simulink model "mmr_air_backup"  (R2019a)
settings: Solver=VariableStepAuto  StartTime=0.0  StopTime=ta  RelTol=1e-1
values from neighbouring files (symbols this model uses):
  g = -9.81    [MMR.m]    (also in MMR_alfa0.m; MMR_alone.m; MMR_hop_zero.m = 9.81)
  Lcol = 0.70    (= 0.7)    [MMR.m]    (also in MMR_alone.m)
  Lhk = 0.28    [MMR.m]    (also in MMR_alfa0.m; MMR_alone.m; MMR_hop_zero.m)
  Lkf = 0.28    [MMR.m]    (also in MMR_alfa0.m; MMR_alone.m; MMR_hop_zero.m)
  M = 15    [MMR.m]    (also in MMR_alfa0.m; MMR_alone.m; MMR_hop_zero.m)
  m = 3    [MMR.m]    (also in MMR_alfa0.m; MMR_alone.m; MMR_hop_zero.m)
  vxfinal = vx( length(vx) )    [MMR.m]    (also in MMR_alfa0.m; MMR_alone.m)
  vxMfinal = vxM( length(vxM) )    [MMR.m]    (also in MMR_alfa0.m; MMR_alone.m)
  vyfinal = vy( length(vy) )    [MMR.m]    (also in MMR_alfa0.m; MMR_alone.m; MMR_hop_zero.m)
  vyMfinal = vyM( length(vyM) )    [MMR.m]    (also in MMR_alfa0.m; MMR_alone.m)
  xfinal = x( length(x) )    [MMR.m]    (also in MMR_alfa0.m; MMR_alone.m)
  xMfinal = xM( length(xM) )    [MMR.m]    (also in MMR_alfa0.m; MMR_alone.m)
  yfinal = y( length(y) )    [MMR.m]    (also in MMR_alfa0.m; MMR_alone.m; MMR_hop_zero.m)
  yMfinal = yM( length(yM) )    [MMR.m]    (also in MMR_alfa0.m; MMR_alone.m)
undefined symbols (not defined in the file or in its folder): magnitude
settings Model: Creator=Jesus  LastModifiedBy=Jesus

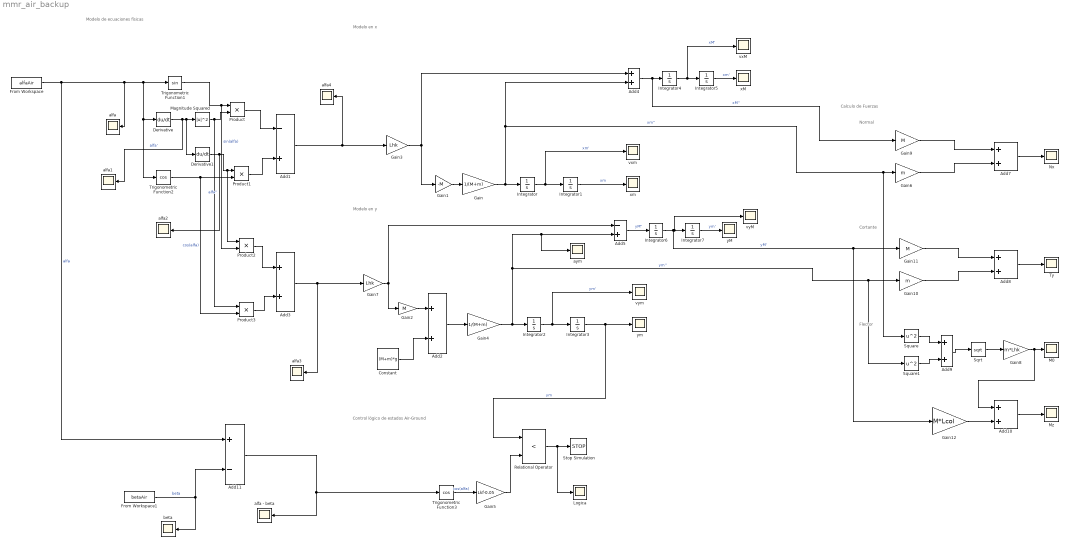
== system mmr_air_backup ==
  note: Control lógico de estados Air-Ground
  note: Modelo de ecuaciones físicas
  note: Modelo en x
  note: Modelo en y
  note: Calculo de Fuerzas
  note: Normal
  note: Cortante
  note: Flector
  Add1 : Sum  Inputs=-+
  Add{2..4,7..10} (7 alike) : Sum
  Add11 : Sum  Inputs=+-
  Add5 : Sum  Inputs=-+
  Constant : Constant  Value=(M+m)*g
  Derivative : Derivative  CoefficientInTFapproximation=1000
  Derivative1 : Derivative  CoefficientInTFapproximation=1000
  From Workspace : FromWorkspace  VariableName=alfaAir  SampleTime=0
  From Workspace1 : FromWorkspace  VariableName=betaAir  SampleTime=0
  Gain : Gain  Gain=1/(M+m)
  Gain1 : Gain  Gain=-M
  Gain10 : Gain  Gain=m
  Gain11 : Gain  Gain=M
  Gain12 : Gain  Gain=M*Lcol
  Gain2 : Gain  Gain=M
  Gain3 : Gain  Gain=Lhk
  Gain4 : Gain  Gain=1/(M+m)
  Gain5 : Gain  Gain=Lkf-0.05
  Gain6 : Gain  Gain=m
  Gain7 : Gain  Gain=Lhk
  Gain8 : Gain  Gain=m*Lhk
  Gain9 : Gain  Gain=M
  Integrator : Integrator  InitialCondition=vxfinal
  Integrator1 : Integrator  InitialCondition=xfinal
  Integrator2 : Integrator  InitialCondition=vyfinal
  Integrator3 : Integrator  InitialCondition=yfinal
  Integrator4 : Integrator  InitialCondition=vxMfinal
  Integrator5 : Integrator  InitialCondition=xMfinal
  Integrator6 : Integrator  InitialCondition=vyMfinal
  Integrator7 : Integrator  InitialCondition=yMfinal
  Logica : Scope
  M0 : Scope
  Magnitude Squared : Math  Operator=magnitude^2  SaturateOnIntegerOverflow=on
  Mz : Scope
  Nx : Scope
  Product{,1..3} (4 alike) : Product
  Relational Operator : RelationalOperator  Operator=<  OutDataTypeStr=boolean  RndMeth=Simplest
  Sqrt : Sqrt  SaturateOnIntegerOverflow=on
  Square : Math  Operator=square  SaturateOnIntegerOverflow=on
  Square1 : Math  Operator=square  SaturateOnIntegerOverflow=on
  Stop Simulation : Stop
  Trigonometric Function1 : Trigonometry
  Trigonometric Function2 : Trigonometry  Operator=cos
  Trigonometric Function3 : Trigonometry  Operator=cos
  Ty : Scope
  alfa{,1..4} (5 alike) : Scope
  alfa - beta : Scope
  aym : Scope
  beta : Scope
  vxM : Scope
  vxm : Scope
  vyM : Scope
  vym : Scope
  xM : Scope
  xm : Scope
  yM : Scope
  ym : Scope
  wires:
  Add2/1 -> Gain4/1
  Constant/1 -> Add2/2
  From Workspace/1 -> Add11/1, alfa/1, Trigonometric Function2/1, Derivative/1, Trigonometric Function1/1  "alfa"
  Add1/1 -> Gain3/1, alfa4/1
  Trigonometric Function1/1 -> Product2/2, Product/1  "sin(alfa)"
  Trigonometric Function2/1 -> Product3/2, Product1/2  "cos(alfa)"
  Derivative1/1 -> alfa2/1, Product1/1, Product2/1  "alfa''"
  Product1/1 -> Add1/2
  Product3/1 -> Add3/2
  Add3/1 -> alfa3/1, Gain7/1
  Product/1 -> Add1/1
  Magnitude Squared/1 -> Product3/1, Product/2
  Product2/1 -> Add3/1
  Derivative/1 -> alfa1/1, Derivative1/1, Magnitude Squared/1  "alfa'"
  Integrator2/1 -> vym/1, Integrator3/1  "ym'"
  Integrator3/1 -> ym/1, Relational Operator/1  "ym"
  Integrator1/1 -> xm/1  "xm"
  Integrator/1 -> vxm/1, Integrator1/1  "xm'"
  Gain1/1 -> Gain/1
  Integrator5/1 -> xM/1  "xm'"
  Gain3/1 -> Add4/1, Gain1/1
  Gain/1 -> Add4/2, Square/1, Gain6/1, Integrator/1  "xm''"
  Add4/1 -> Gain9/1, Integrator4/1  "xM''"
  Integrator4/1 -> vxM/1, Integrator5/1  "xM'"
  Gain2/1 -> Add2/1
  Gain7/1 -> Gain2/1, Add5/1
  Add5/1 -> Integrator6/1  "yM''"
  Integrator6/1 -> Gain12/1, Gain11/1, vyM/1, Integrator7/1  "yM'"
  Gain4/1 -> Add5/2, aym/1, Square1/1, Gain10/1, Integrator2/1  "ym''"
  Integrator7/1 -> yM/1  "ym'"
  Relational Operator/1 -> Logica/1, Stop Simulation/1
  Gain5/1 -> Relational Operator/2
  Trigonometric Function3/1 -> Gain5/1  "cos(alfa)"
  Add11/1 -> alfa - beta/1, Trigonometric Function3/1
  From Workspace1/1 -> Add11/2, beta/1  "beta"
  Gain8/1 -> Add10/1, M0/1
  Add7/1 -> Nx/1
  Gain9/1 -> Add7/1
  Gain6/1 -> Add7/2
  Gain11/1 -> Add8/1
  Gain10/1 -> Add8/2
  Add8/1 -> Ty/1
  Square/1 -> Add9/1
  Square1/1 -> Add9/2
  Add9/1 -> Sqrt/1
  Sqrt/1 -> Gain8/1
  Add10/1 -> Mz/1
  Gain12/1 -> Add10/2
